simulink model "Basic"  (R2022b)
settings: configuration reference "ERT" (kept outside this file)
PreLoadFcn:
  | %rtwdemo_pmsmfoc_data
StartFcn:
  | %clear executionProfile
StopFcn:
  | %try
  | %  AddExecutionProfileToDataInspector();
  | %end
undefined symbols (not defined in the file or in its folder): bSetOfsAlMdl_C, bSetOfsAlOvrd_C, bUseFrqStrSyntMdl_C, bUseFrqStrSyntOvrd_C, ctrlModeMdl_C, ctrlModeOvrd_C, cTrqSlopeMaxMdl_C, cTrqSlopeMaxOvrd_C, flgInvrCanActvnCmdMdl_C, flgInvrCanActvnCmdOvrd_C, FrqStrSetPMdl_C, FrqStrSetPOvrd_C, IdcMaxMdl_C, IdcMaxOvrd_C, iDCmdMdl_C, iDCmdOvrd_C, IdcMinMdl_C, IdcMinOvrd_C, iQCmdMdl_C, iQCmdOvrd_C, IsSetPMdl_C, IsSetPOvrd_C, kDmpMdl_C, kDmpOvrd_C, KpHighMdl_C, KpHighOvrd_C, KpLowMdl_C, KpLowOvrd_C, NDeltaBoundMdl_C, NDeltaBoundOvrd_C, NSetPMdl_C, NSetPOvrd_C, OfsAlMdl_C, OfsAlOvrd_C, PumpCtlMdl_C, PumpCtlOvrd_C, stDstCReqMdl_C, stDstCReqOvrd_C, stHvbMaiRlyMdl_C, stHvbMaiRlyOvrd_C, stModeReqMdl_C, stModeReqOvrd_C, TrqDmpLimMdl_C, TrqDmpLimOvrd_C, TrqDmpMaxMdl_C, TrqDmpMaxOvrd_C, TrqMaxMdl_C, TrqMaxOvrd_C, TrqMinMdl_C, TrqMinOvrd_C, TrqPAmaxMdl_C, TrqPAmaxOvrd_C, TrqPAminMdl_C, TrqPAminOvrd_C, TrqSetPMdl_C, TrqSetPOvrd_C, Ts_10ms, Ts_1ms, uAlphaCmdMdl_C, uAlphaCmdOvrd_C ... (+12)
settings Model: Creator=The MathWorks, Inc.  LastModifiedBy=M00039784
settings ConfigSetRef: SourceName=ERT  SourceLocation=Base Workspace

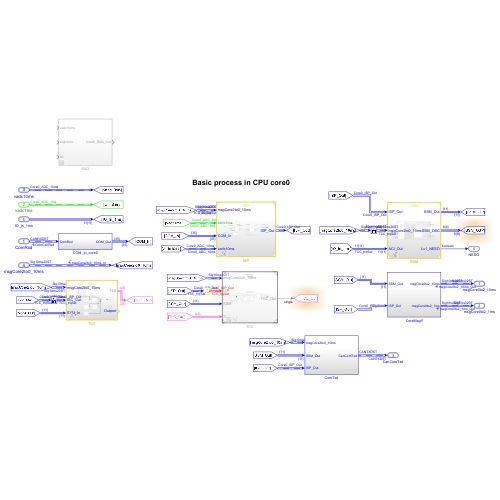
[thumbnail: Simulink's stored preview of the top-level diagram]
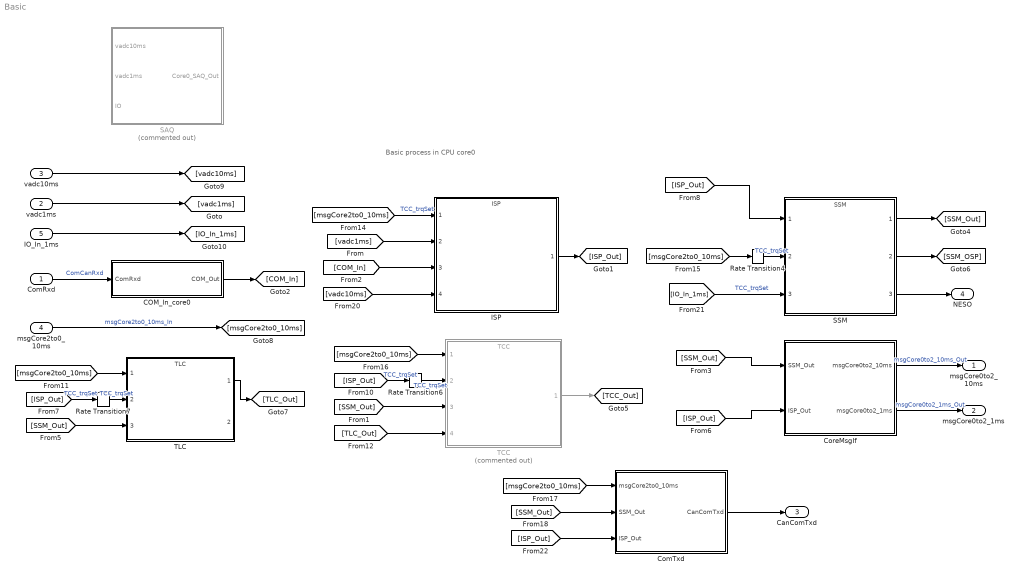
== system Basic ==
  note: Basic process in CPU core0
  ComRxd : Inport  OutDataTypeStr=Bus: CANRXDST  SampleTime=Ts_10ms  BusOutputAsStruct=on
  vadc1ms : Inport  Port=2  OutDataTypeStr=Bus: Core0_ADC_1ms  SampleTime=Ts_1ms  BusOutputAsStruct=on
  vadc10ms : Inport  Port=3  OutDataTypeStr=Bus: Core0_ADC_10ms  SampleTime=Ts_10ms  BusOutputAsStruct=on
  msgCore2to0_10ms : Inport  Port=4  OutDataTypeStr=Bus: Sig10ms20ST  SampleTime=Ts_10ms  BusOutputAsStruct=on
  IO_In_1ms : Inport  Port=5  OutDataTypeStr=Bus: IO_In_1ms
  COM_In_core0 : Subsystem
  ComTxd : Subsystem
  CoreMsgIf : Subsystem
  ISP : ModelReference  ModelNameDialog=ISP.slx  SimulationMode=Normal  ModelReferenceVersion=1.15
  Rate Transition4 : RateTransition  Deterministic=off
  Rate Transition6 : RateTransition  Deterministic=off
  Rate Transition7 : RateTransition  Deterministic=off
  SAQ : Subsystem  Commented=on
  SSM : ModelReference  ModelNameDialog=SSM.slx  SimulationMode=Normal  ModelReferenceVersion=1.14
  TCC : ModelReference  Commented=on  ModelNameDialog=TCC.slx  SimulationMode=Normal  ModelReferenceVersion=1.4
  TLC : ModelReference  ModelNameDialog=TLC.slx  SimulationMode=Normal  ModelReferenceVersion=1.7
  msgCore0to2_10ms : Outport  OutDataTypeStr=Bus: Sig10ms02ST  VectorParamsAs1DForOutWhenUnconnected=off
  msgCore0to2_1ms : Outport  Port=2  OutDataTypeStr=Bus: Sig1ms02ST  VectorParamsAs1DForOutWhenUnconnected=off
  CanComTxd : Outport  Port=3  OutDataTypeStr=Bus: CANTXDST  SampleTime=Ts_10ms  VectorParamsAs1DForOutWhenUnconnected=off
  NESO : Outport  Port=4  SampleTime=Ts_10ms  VectorParamsAs1DForOutWhenUnconnected=off
  wires:
  ComRxd/1 -> COM_In_core0/1(ComRxd)  "ComCanRxd"
  COM_In_core0/1(COM_Out) -> [COM_In]
  SSM/1 -> [SSM_Out]
  [SSM_Out] -> TLC/3
  TLC/1 -> [TLC_Out]
  [TLC_Out] -> TCC/4
  [SSM_Out] -> TCC/3
  TCC/1 -> [TCC_Out]
  [COM_In] -> ISP/3
  [SSM_Out] -> CoreMsgIf/1(SSM_Out)
  [ISP_Out] -> CoreMsgIf/2(ISP_Out)
  CoreMsgIf/1(msgCore0to2_10ms) -> msgCore0to2_10ms/1  "msgCore0to2_10ms_Out"
  CoreMsgIf/2(msgCore0to2_1ms) -> msgCore0to2_1ms/1  "msgCore0to2_1ms_Out"
  SSM/2 -> [SSM_OSP]
  msgCore2to0_10ms/1 -> [msgCore2to0_10ms]  "msgCore2to0_10ms_In"
  [msgCore2to0_10ms] -> TLC/1
  [msgCore2to0_10ms] -> Rate Transition4/1
  [msgCore2to0_10ms] -> TCC/1
  SSM/3 -> NESO/1
  [msgCore2to0_10ms] -> ComTxd/1(msgCore2to0_10ms)
  [SSM_Out] -> ComTxd/2(SSM_Out)
  [ISP_Out] -> ComTxd/3(ISP_Out)
  ComTxd/1(CanComTxd) -> CanComTxd/1
  [msgCore2to0_10ms] -> ISP/1  "TCC_trqSet"
  [ISP_Out] -> Rate Transition7/1  "TCC_trqSet"
  [ISP_Out] -> Rate Transition6/1  "TCC_trqSet"
  ISP/1 -> [ISP_Out]
  Rate Transition4/1 -> SSM/2  "TCC_trqSet"
  Rate Transition6/1 -> TCC/2  "TCC_trqSet"
  Rate Transition7/1 -> TLC/2  "TCC_trqSet"
  vadc10ms/1 -> [vadc10ms]
  IO_In_1ms/1 -> [IO_In_1ms]
  vadc1ms/1 -> [vadc1ms]
  [vadc1ms] -> ISP/2
  [vadc10ms] -> ISP/4
  [ISP_Out] -> SSM/1
  [IO_In_1ms] -> SSM/3  "TCC_trqSet"

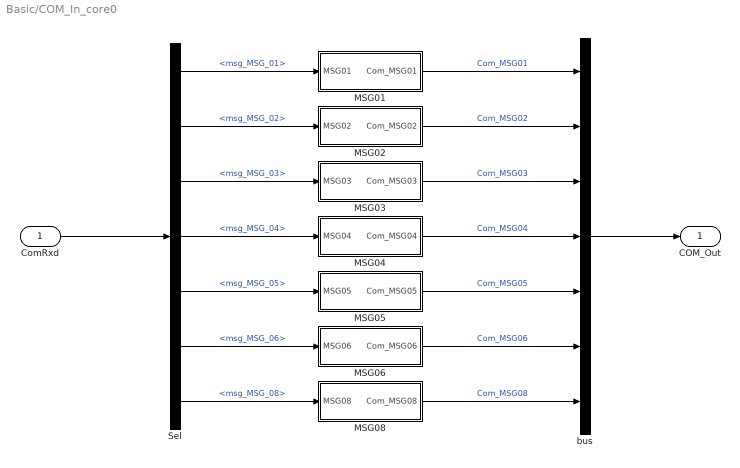
== system Basic/COM_In_core0 ==
  ComRxd : Inport  OutDataTypeStr=Bus: CANRXDST
  MSG01 : Subsystem
  MSG02 : Subsystem
  MSG03 : Subsystem
  MSG04 : Subsystem
  MSG05 : Subsystem
  MSG06 : Subsystem
  MSG08 : Subsystem
  Sel : BusSelector  OutputSignals=msg_MSG_01,msg_MSG_02,msg_MSG_03,msg_MSG_04,msg_MSG_05,msg_MSG_06,msg_MSG_08
  bus : BusCreator  Inputs=7  OutDataTypeStr=Bus: Core0_COM_Out
  COM_Out : Outport  OutDataTypeStr=Bus: Core0_COM_Out  VectorParamsAs1DForOutWhenUnconnected=off
  wires:
  ComRxd/1 -> Sel/1
  bus/1 -> COM_Out/1
  Sel/1 -> MSG01/1(MSG01)  "<msg_MSG_01>"
  MSG01/1(Com_MSG01) -> bus/1  "Com_MSG01"
  Sel/2 -> MSG02/1(MSG02)  "<msg_MSG_02>"
  MSG02/1(Com_MSG02) -> bus/2  "Com_MSG02"
  Sel/3 -> MSG03/1(MSG03)  "<msg_MSG_03>"
  MSG03/1(Com_MSG03) -> bus/3  "Com_MSG03"
  Sel/4 -> MSG04/1(MSG04)  "<msg_MSG_04>"
  MSG04/1(Com_MSG04) -> bus/4  "Com_MSG04"
  Sel/5 -> MSG05/1(MSG05)  "<msg_MSG_05>"
  MSG05/1(Com_MSG05) -> bus/5  "Com_MSG05"
  Sel/6 -> MSG06/1(MSG06)  "<msg_MSG_06>"
  MSG06/1(Com_MSG06) -> bus/6  "Com_MSG06"
  Sel/7 -> MSG08/1(MSG08)  "<msg_MSG_08>"
  MSG08/1(Com_MSG08) -> bus/7  "Com_MSG08"

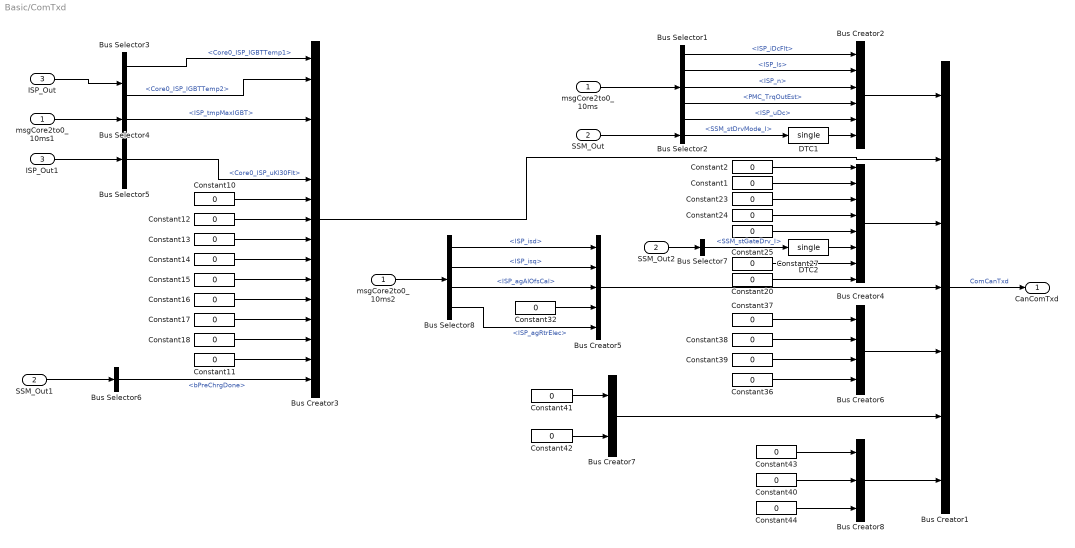
== system Basic/ComTxd ==
  msgCore2to0_10ms : Inport  OutDataTypeStr=Bus: Sig10ms20ST
  SSM_Out : Inport  Port=2  OutDataTypeStr=Bus: Core0_SSM_Out
  ISP_Out : Inport  Port=3  OutDataTypeStr=Bus: Core0_ISP_Out
  Bus Creator1 : BusCreator  Inputs=7  OutDataTypeStr=Bus: CANTXDST  NonVirtualBus=on
  Bus Creator2 : BusCreator  Inputs=6  OutDataTypeStr=Bus: msg_EM_01
  Bus Creator3 : BusCreator  Inputs=17  OutDataTypeStr=Bus: msg_EM_02
  Bus Creator4 : BusCreator  Inputs=8  OutDataTypeStr=Bus: msg_EM_03
  Bus Creator5 : BusCreator  Inputs=5  OutDataTypeStr=Bus: msg_EM_04
  Bus Creator6 : BusCreator  Inputs=4  OutDataTypeStr=Bus: msg_EM_05
  Bus Creator7 : BusCreator  Inputs=2  OutDataTypeStr=Bus: msg_EM_06
  Bus Creator8 : BusCreator  Inputs=3  OutDataTypeStr=Bus: msg_EM_07
  Bus Selector1 : BusSelector  OutputSignals=ISP_iDcFlt,ISP_Is,ISP_n,PMC_TrqOutEst,ISP_uDc
  Bus Selector2 : BusSelector  OutputSignals=SSM_stDrvMode_I
  Bus Selector3 : BusSelector  OutputSignals=Core0_ISP_AnaOut.Core0_ISP_tInvx.Core0_tInv.Core0_ISP_IGBTTemp1,Core0_ISP_AnaOut.Core0_ISP_tInvx.Core0_tInv.Core0_ISP_IGBTTemp2
  Bus Selector4 : BusSelector  OutputSignals=ISP_tmpMaxIGBT
  Bus Selector5 : BusSelector  OutputSignals=Core0_ISP_AnaOut.Core0_ISP_uKl30Flt
  Bus Selector6 : BusSelector  OutputSignals=bPreChrgDone
  Bus Selector7 : BusSelector  OutputSignals=SSM_stGateDrv_I
  Bus Selector8 : BusSelector  OutputSignals=ISP_isd,ISP_isq,ISP_agAlOfsCal,ISP_agRtrElec
  Constant{1..2,20,23..25,27,32,36..44} (17 alike) : Constant  Value=0  OutDataTypeStr=single
  Constant{10..18} (9 alike) : Constant  Value=0  OutDataTypeStr=boolean
  DTC1 : DataTypeConversion  OutDataTypeStr=single  SaturateOnIntegerOverflow=off  RndMeth=Floor
  DTC2 : DataTypeConversion  OutDataTypeStr=single  SaturateOnIntegerOverflow=off  RndMeth=Floor
  ISP_Out1 : InportShadow  Port=3  OutDataTypeStr=Bus: Core0_ISP_Out
  SSM_Out1 : InportShadow  Port=2  OutDataTypeStr=Bus: Core0_SSM_Out
  SSM_Out2 : InportShadow  Port=2  OutDataTypeStr=Bus: Core0_SSM_Out
  msgCore2to0_10ms1 : InportShadow  OutDataTypeStr=Bus: Sig10ms20ST
  msgCore2to0_10ms2 : InportShadow  OutDataTypeStr=Bus: Sig10ms20ST
  CanComTxd : Outport  OutDataTypeStr=Bus: CANTXDST  SampleTime=Ts_10ms  VectorParamsAs1DForOutWhenUnconnected=off
  wires:
  Bus Creator1/1 -> CanComTxd/1  "ComCanTxd"
  msgCore2to0_10ms/1 -> Bus Selector1/1
  Bus Creator2/1 -> Bus Creator1/1
  Bus Selector1/1 -> Bus Creator2/1  "<ISP_iDcFlt>"
  Bus Selector1/2 -> Bus Creator2/2  "<ISP_Is>"
  Bus Selector1/3 -> Bus Creator2/3  "<ISP_n>"
  Bus Creator3/1 -> Bus Creator1/2
  Bus Creator4/1 -> Bus Creator1/3
  Bus Creator5/1 -> Bus Creator1/4
  Bus Creator6/1 -> Bus Creator1/5
  Bus Creator7/1 -> Bus Creator1/6
  Bus Creator8/1 -> Bus Creator1/7
  Bus Selector2/1 -> DTC1/1  "<SSM_stDrvMode_I>"
  Bus Selector3/1 -> Bus Creator3/1  "<Core0_ISP_IGBTTemp1>"
  Bus Selector3/2 -> Bus Creator3/2  "<Core0_ISP_IGBTTemp2>"
  Bus Selector4/1 -> Bus Creator3/4  "<ISP_tmpMaxIGBT>"
  Constant10/1 -> Bus Creator3/8
  Constant18/1 -> Bus Creator3/15
  Constant16/1 -> Bus Creator3/13
  Constant11/1 -> Bus Creator3/16
  Constant12/1 -> Bus Creator3/9
  Constant13/1 -> Bus Creator3/10
  Constant14/1 -> Bus Creator3/11
  Constant15/1 -> Bus Creator3/12
  Constant17/1 -> Bus Creator3/14
  Bus Selector6/1 -> Bus Creator3/17  "<bPreChrgDone>"
  Constant2/1 -> Bus Creator4/1
  Constant1/1 -> Bus Creator4/2
  Constant23/1 -> Bus Creator4/3
  Constant24/1 -> Bus Creator4/4
  Constant25/1 -> Bus Creator4/5
  DTC2/1 -> Bus Creator4/6
  Constant27/1 -> Bus Creator4/7
  Constant20/1 -> Bus Creator4/8
  Bus Selector8/1 -> Bus Creator5/1  "<ISP_isd>"
  Bus Selector8/3 -> Bus Creator5/3  "<ISP_agAlOfsCal>"
  Bus Selector8/2 -> Bus Creator5/2  "<ISP_isq>"
  Bus Selector8/4 -> Bus Creator5/5  "<ISP_agRtrElec>"
  Constant32/1 -> Bus Creator5/4
  Constant37/1 -> Bus Creator6/1
  Constant38/1 -> Bus Creator6/2
  Constant39/1 -> Bus Creator6/3
  Constant36/1 -> Bus Creator6/4
  Constant41/1 -> Bus Creator7/1
  Constant42/1 -> Bus Creator7/2
  Constant44/1 -> Bus Creator8/3
  Constant40/1 -> Bus Creator8/2
  Constant43/1 -> Bus Creator8/1
  Bus Selector1/4 -> Bus Creator2/4  "<PMC_TrqOutEst>"
  Bus Selector1/5 -> Bus Creator2/5  "<ISP_uDc>"
  SSM_Out/1 -> Bus Selector2/1
  DTC1/1 -> Bus Creator2/6
  ISP_Out/1 -> Bus Selector3/1
  msgCore2to0_10ms1/1 -> Bus Selector4/1
  ISP_Out1/1 -> Bus Selector5/1
  SSM_Out1/1 -> Bus Selector6/1
  SSM_Out2/1 -> Bus Selector7/1
  Bus Selector7/1 -> DTC2/1  "<SSM_stGateDrv_I>"
  msgCore2to0_10ms2/1 -> Bus Selector8/1
  Bus Selector5/1 -> Bus Creator3/7  "<Core0_ISP_uKl30Flt>"

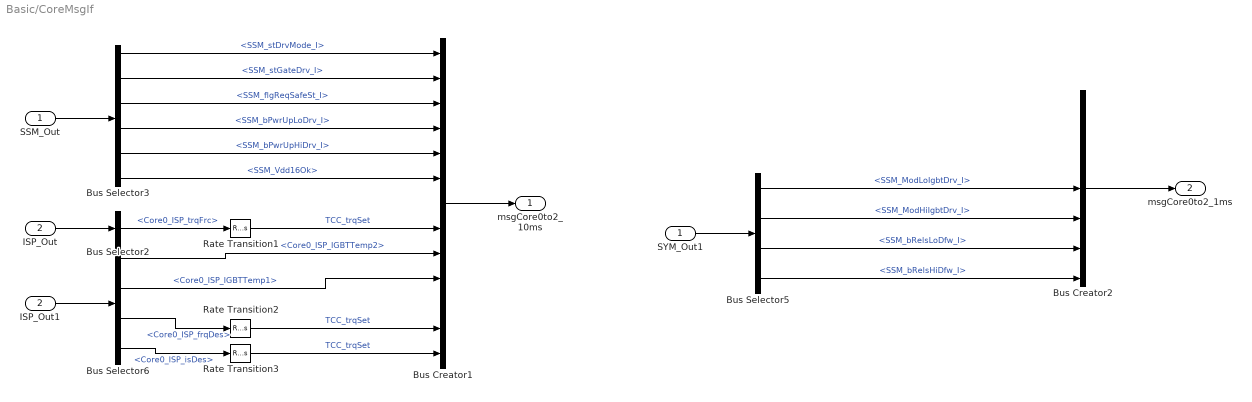
== system Basic/CoreMsgIf ==
  SSM_Out : Inport  OutDataTypeStr=Bus: Core0_SSM_Out
  ISP_Out : Inport  Port=2  OutDataTypeStr=Bus: Core0_ISP_Out
  Bus Creator1 : BusCreator  Inputs=13  OutDataTypeStr=Bus: Sig10ms02ST  NonVirtualBus=on
      settings: InheritFromInputs=off
  Bus Creator2 : BusCreator  Inputs=7  OutDataTypeStr=Bus: Sig1ms02ST  NonVirtualBus=on
      settings: InheritFromInputs=off
  Bus Selector2 : BusSelector  OutputSignals=Core0_ISP_ComCmd.Core0_ISP_trqx.Core0_ISP_trqFrc
  Bus Selector3 : BusSelector  OutputSignals=SSM_stDrvMode_I,SSM_stGateDrv_I,SSM_flgReqSafeSt_I,SSM_bPwrUpLoDrv_I,SSM_bPwrUpHiDrv_I,SSM_Vdd16Ok
  Bus Selector5 : BusSelector  OutputSignals=SSM_ModLoIgbtDrv_I,SSM_ModHiIgbtDrv_I,SSM_bRelsLoDfw_I,SSM_bRelsHiDfw_I
  Bus Selector6 : BusSelector  OutputSignals=Core0_ISP_AnaOut.Core0_ISP_tInvx.Core0_tInv.Core0_ISP_IGBTTemp2,Core0_ISP_AnaOut.Core0_ISP_tInvx.Core0_tInv.Core0_ISP_IGBTTemp1,Core0_ISP_ComCmd.Core0_ISP_cmdx.Core0_ISP_frqDes,Core0_ISP_ComCmd.Core0_ISP_cmdx.Core0_ISP_isDes
  ISP_Out1 : InportShadow  Port=2  OutDataTypeStr=Bus: Core0_ISP_Out
  Rate Transition1 : RateTransition  Deterministic=off  OutPortSampleTime=Ts_10ms
  Rate Transition2 : RateTransition  Deterministic=off  OutPortSampleTime=Ts_10ms
  Rate Transition3 : RateTransition  Deterministic=off  OutPortSampleTime=Ts_10ms
  SYM_Out1 : InportShadow  OutDataTypeStr=Bus: Core0_SSM_Out
  msgCore0to2_10ms : Outport  OutDataTypeStr=Bus: Sig10ms02ST  VectorParamsAs1DForOutWhenUnconnected=off
  msgCore0to2_1ms : Outport  Port=2  OutDataTypeStr=Bus: Sig1ms02ST  VectorParamsAs1DForOutWhenUnconnected=off
  wires:
  Bus Selector3/1 -> Bus Creator1/1  "<SSM_stDrvMode_I>"
  Bus Selector3/2 -> Bus Creator1/2  "<SSM_stGateDrv_I>"
  Bus Creator1/1 -> msgCore0to2_10ms/1
  SSM_Out/1 -> Bus Selector3/1
  Bus Selector2/1 -> Rate Transition1/1  "<Core0_ISP_trqFrc>"
  Bus Selector3/3 -> Bus Creator1/3  "<SSM_flgReqSafeSt_I>"
  ISP_Out/1 -> Bus Selector2/1
  Bus Creator2/1 -> msgCore0to2_1ms/1
  Bus Selector3/4 -> Bus Creator1/4  "<SSM_bPwrUpLoDrv_I>"
  Bus Selector3/5 -> Bus Creator1/5  "<SSM_bPwrUpHiDrv_I>"
  SYM_Out1/1 -> Bus Selector5/1
  Bus Selector5/1 -> Bus Creator2/4  "<SSM_ModLoIgbtDrv_I>"
  Bus Selector5/2 -> Bus Creator2/5  "<SSM_ModHiIgbtDrv_I>"
  Bus Selector5/3 -> Bus Creator2/6  "<SSM_bRelsLoDfw_I>"
  Bus Selector5/4 -> Bus Creator2/7  "<SSM_bRelsHiDfw_I>"
  ISP_Out1/1 -> Bus Selector6/1
  Bus Selector6/1 -> Bus Creator1/9  "<Core0_ISP_IGBTTemp2>"
  Bus Selector6/2 -> Bus Creator1/10  "<Core0_ISP_IGBTTemp1>"
  Bus Selector3/6 -> Bus Creator1/6  "<SSM_Vdd16Ok>"
  Bus Selector6/3 -> Rate Transition2/1  "<Core0_ISP_frqDes>"
  Bus Selector6/4 -> Rate Transition3/1  "<Core0_ISP_isDes>"
  Rate Transition1/1 -> Bus Creator1/8  "TCC_trqSet"
  Rate Transition2/1 -> Bus Creator1/12  "TCC_trqSet"
  Rate Transition3/1 -> Bus Creator1/13  "TCC_trqSet"

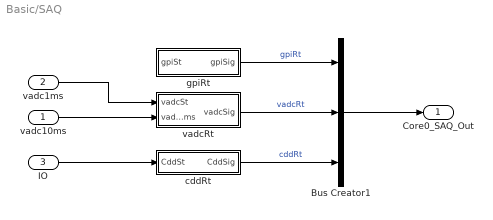
== system Basic/SAQ ==
  vadc10ms : Inport  OutDataTypeStr=Bus: Core0_ADC_10ms
  vadc1ms : Inport  Port=2  OutDataTypeStr=Bus: Core0_ADC_1ms
  IO : Inport  Port=3  OutDataTypeStr=Bus: IO_In_1ms
  Bus Creator1 : BusCreator  Inputs=3  OutDataTypeStr=Bus: Core0_SAQ_Out  NonVirtualBus=on
  cddRt : Subsystem
  gpiRt : Subsystem
  vadcRt : Subsystem
  Core0_SAQ_Out : Outport  OutDataTypeStr=Bus: Core0_SAQ_Out  VectorParamsAs1DForOutWhenUnconnected=off
      settings: AttributesFormatString=Disable Action: %<OutputWhenDisabled>
  wires:
  Bus Creator1/1 -> Core0_SAQ_Out/1
  gpiRt/1(gpiSig) -> Bus Creator1/1  "gpiRt"
  vadc10ms/1 -> vadcRt/2(vadc10ms)
  vadc1ms/1 -> vadcRt/1(vadcSt)
  vadcRt/1(vadcSig) -> Bus Creator1/2  "vadcRt"
  IO/1 -> cddRt/1(CddSt)
  cddRt/1(CddSig) -> Bus Creator1/3  "cddRt"

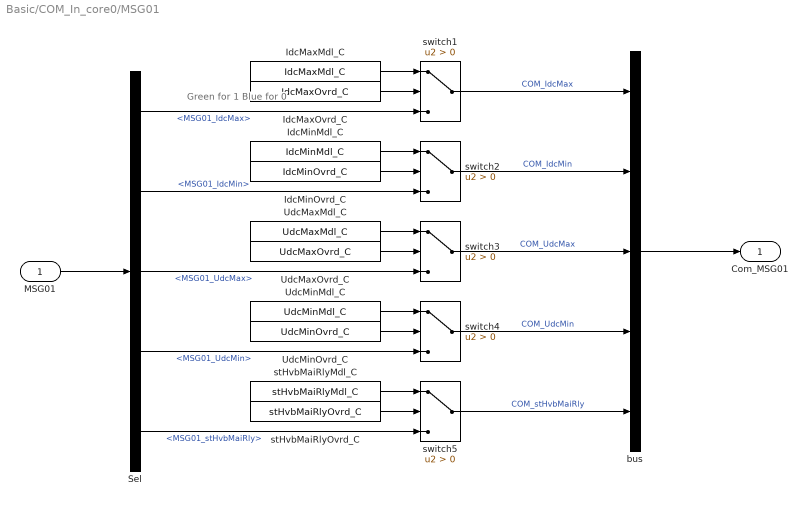
== system Basic/COM_In_core0/MSG01 ==
  note: Green  for 1
      | Blue  for 0
  MSG01 : Inport
  IdcMaxMdl_C : Constant  Value=IdcMaxMdl_C
      mask Display:
      | tmpx = get_param(gcbh,'Value');
      | a= evalin('base',[tmpx,'.Value;']);
      | disp([tmpx,': ',num2str(a)]);
  IdcMaxOvrd_C : Constant  Value=IdcMaxOvrd_C
      mask Display:
      | tmpx = get_param(gcbh,'Value');
      | a= evalin('base',[tmpx,'.Value;']);
      | if a==0
      |     color('blue');
      | else
      |     color('green');
      | end
      | disp([tmpx,': ',num2str(a)]);
  IdcMinMdl_C : Constant  Value=IdcMinMdl_C
      mask Display:
      | tmpx = get_param(gcbh,'Value');
      | a= evalin('base',[tmpx,'.Value;']);
      | disp([tmpx,': ',num2str(a)]);
  IdcMinOvrd_C : Constant  Value=IdcMinOvrd_C
      mask Display:
      | tmpx = get_param(gcbh,'Value');
      | a= evalin('base',[tmpx,'.Value;']);
      | if a==0
      |     color('red');
      | else
      |     color('green');
      | end
      | disp([tmpx,': ',num2str(a)]);
  Sel : BusSelector  OutputSignals=MSG01_IdcMax,MSG01_IdcMin,MSG01_UdcMax,MSG01_UdcMin,MSG01_stHvbMaiRly
  UdcMaxMdl_C : Constant  Value=UdcMaxMdl_C
      mask Display:
      | tmpx = get_param(gcbh,'Value');
      | a= evalin('base',[tmpx,'.Value;']);
      | disp([tmpx,': ',num2str(a)]);
  UdcMaxOvrd_C : Constant  Value=UdcMaxOvrd_C
      mask Display:
      | tmpx = get_param(gcbh,'Value');
      | a= evalin('base',[tmpx,'.Value;']);
      | if a==0
      |     color('blue');
      | else
      |     color('green');
      | end
      | disp([tmpx,': ',num2str(a)]);
  UdcMinMdl_C : Constant  Value=UdcMinMdl_C
      mask Display:
      | tmpx = get_param(gcbh,'Value');
      | a= evalin('base',[tmpx,'.Value;']);
      | disp([tmpx,': ',num2str(a)]);
  UdcMinOvrd_C : Constant  Value=UdcMinOvrd_C
      mask Display:
      | tmpx = get_param(gcbh,'Value');
      | a= evalin('base',[tmpx,'.Value;']);
      | if a==0
      |     color('blue');
      | else
      |     color('green');
      | end
      | disp([tmpx,': ',num2str(a)]);
  bus : BusCreator  Inputs=5
  stHvbMaiRlyMdl_C : Constant  Value=stHvbMaiRlyMdl_C
      mask Display:
      | tmpx = get_param(gcbh,'Value');
      | a= evalin('base',[tmpx,'.Value;']);
      | disp([tmpx,': ',num2str(a)]);
  stHvbMaiRlyOvrd_C : Constant  Value=stHvbMaiRlyOvrd_C
      mask Display:
      | tmpx = get_param(gcbh,'Value');
      | a= evalin('base',[tmpx,'.Value;']);
      | if a==0
      |     color('blue');
      | else
      |     color('green');
      | end
      | disp([tmpx,': ',num2str(a)]);
  switch{1..5} (5 alike) : Switch  Criteria=u2 > Threshold  SaturateOnIntegerOverflow=off  InputSameDT=off
  Com_MSG01 : Outport  VectorParamsAs1DForOutWhenUnconnected=off
  wires:
  MSG01/1 -> Sel/1
  bus/1 -> Com_MSG01/1
  IdcMaxOvrd_C/1 -> switch1/2
  IdcMaxMdl_C/1 -> switch1/1
  switch1/1 -> bus/1  "COM_IdcMax"
  Sel/1 -> switch1/3  "<MSG01_IdcMax>"
  IdcMinOvrd_C/1 -> switch2/2
  IdcMinMdl_C/1 -> switch2/1
  switch2/1 -> bus/2  "COM_IdcMin"
  Sel/2 -> switch2/3  "<MSG01_IdcMin>"
  UdcMaxOvrd_C/1 -> switch3/2
  UdcMaxMdl_C/1 -> switch3/1
  switch3/1 -> bus/3  "COM_UdcMax"
  Sel/3 -> switch3/3  "<MSG01_UdcMax>"
  UdcMinOvrd_C/1 -> switch4/2
  UdcMinMdl_C/1 -> switch4/1
  switch4/1 -> bus/4  "COM_UdcMin"
  Sel/4 -> switch4/3  "<MSG01_UdcMin>"
  stHvbMaiRlyOvrd_C/1 -> switch5/2
  stHvbMaiRlyMdl_C/1 -> switch5/1
  switch5/1 -> bus/5  "COM_stHvbMaiRly"
  Sel/5 -> switch5/3  "<MSG01_stHvbMaiRly>"

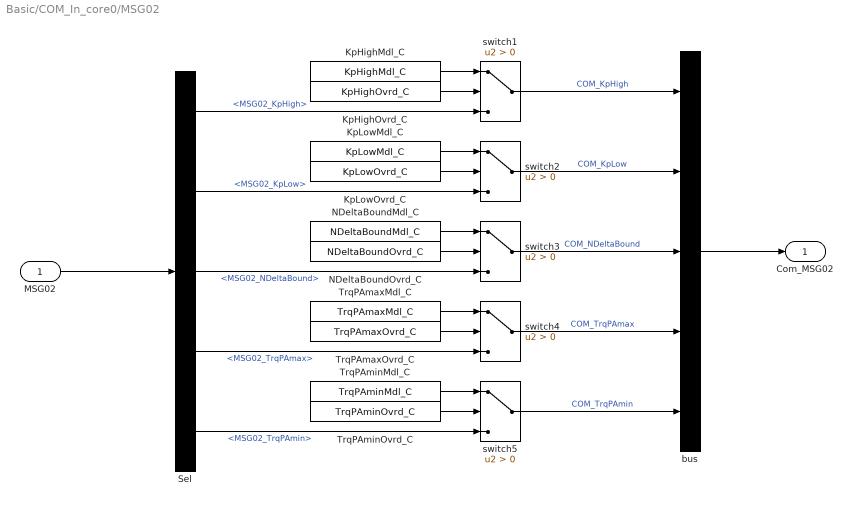
== system Basic/COM_In_core0/MSG02 ==
  MSG02 : Inport
  KpHighMdl_C : Constant  Value=KpHighMdl_C
      mask Display:
      | tmpx = get_param(gcbh,'Value');
      | a= evalin('base',[tmpx,'.Value;']);
      | disp([tmpx,': ',num2str(a)]);
  KpHighOvrd_C : Constant  Value=KpHighOvrd_C
      mask Display:
      | tmpx = get_param(gcbh,'Value');
      | a= evalin('base',[tmpx,'.Value;']);
      | if a==0
      |     color('blue');
      | else
      |     color('green');
      | end
      | disp([tmpx,': ',num2str(a)]);
  KpLowMdl_C : Constant  Value=KpLowMdl_C
      mask Display:
      | tmpx = get_param(gcbh,'Value');
      | a= evalin('base',[tmpx,'.Value;']);
      | disp([tmpx,': ',num2str(a)]);
  KpLowOvrd_C : Constant  Value=KpLowOvrd_C
      mask Display:
      | tmpx = get_param(gcbh,'Value');
      | a= evalin('base',[tmpx,'.Value;']);
      | if a==0
      |     color('blue');
      | else
      |     color('green');
      | end
      | disp([tmpx,': ',num2str(a)]);
  NDeltaBoundMdl_C : Constant  Value=NDeltaBoundMdl_C
      mask Display:
      | tmpx = get_param(gcbh,'Value');
      | a= evalin('base',[tmpx,'.Value;']);
      | disp([tmpx,': ',num2str(a)]);
  NDeltaBoundOvrd_C : Constant  Value=NDeltaBoundOvrd_C
      mask Display:
      | tmpx = get_param(gcbh,'Value');
      | a= evalin('base',[tmpx,'.Value;']);
      | if a==0
      |     color('blue');
      | else
      |     color('green');
      | end
      | disp([tmpx,': ',num2str(a)]);
  Sel : BusSelector  OutputSignals=MSG02_KpHigh,MSG02_KpLow,MSG02_NDeltaBound,MSG02_TrqPAmax,MSG02_TrqPAmin
  TrqPAmaxMdl_C : Constant  Value=TrqPAmaxMdl_C
      mask Display:
      | tmpx = get_param(gcbh,'Value');
      | a= evalin('base',[tmpx,'.Value;']);
      | disp([tmpx,': ',num2str(a)]);
  TrqPAmaxOvrd_C : Constant  Value=TrqPAmaxOvrd_C
      mask Display:
      | tmpx = get_param(gcbh,'Value');
      | a= evalin('base',[tmpx,'.Value;']);
      | if a==0
      |     color('blue');
      | else
      |     color('green');
      | end
      | disp([tmpx,': ',num2str(a)]);
  TrqPAminMdl_C : Constant  Value=TrqPAminMdl_C
      mask Display:
      | tmpx = get_param(gcbh,'Value');
      | a= evalin('base',[tmpx,'.Value;']);
      | disp([tmpx,': ',num2str(a)]);
  TrqPAminOvrd_C : Constant  Value=TrqPAminOvrd_C
      mask Display:
      | tmpx = get_param(gcbh,'Value');
      | a= evalin('base',[tmpx,'.Value;']);
      | if a==0
      |     color('blue');
      | else
      |     color('green');
      | end
      | disp([tmpx,': ',num2str(a)]);
  bus : BusCreator  Inputs=5  OutDataTypeStr=Bus: Com_MSG02
  switch{1..5} (5 alike) : Switch  Criteria=u2 > Threshold  SaturateOnIntegerOverflow=off  InputSameDT=off
  Com_MSG02 : Outport  VectorParamsAs1DForOutWhenUnconnected=off
  wires:
  MSG02/1 -> Sel/1
  bus/1 -> Com_MSG02/1
  KpHighOvrd_C/1 -> switch1/2
  KpHighMdl_C/1 -> switch1/1
  switch1/1 -> bus/1  "COM_KpHigh"
  Sel/1 -> switch1/3  "<MSG02_KpHigh>"
  KpLowOvrd_C/1 -> switch2/2
  KpLowMdl_C/1 -> switch2/1
  switch2/1 -> bus/2  "COM_KpLow"
  Sel/2 -> switch2/3  "<MSG02_KpLow>"
  NDeltaBoundOvrd_C/1 -> switch3/2
  NDeltaBoundMdl_C/1 -> switch3/1
  switch3/1 -> bus/3  "COM_NDeltaBound"
  Sel/3 -> switch3/3  "<MSG02_NDeltaBound>"
  TrqPAmaxOvrd_C/1 -> switch4/2
  TrqPAmaxMdl_C/1 -> switch4/1
  switch4/1 -> bus/4  "COM_TrqPAmax"
  Sel/4 -> switch4/3  "<MSG02_TrqPAmax>"
  TrqPAminOvrd_C/1 -> switch5/2
  TrqPAminMdl_C/1 -> switch5/1
  switch5/1 -> bus/5  "COM_TrqPAmin"
  Sel/5 -> switch5/3  "<MSG02_TrqPAmin>"

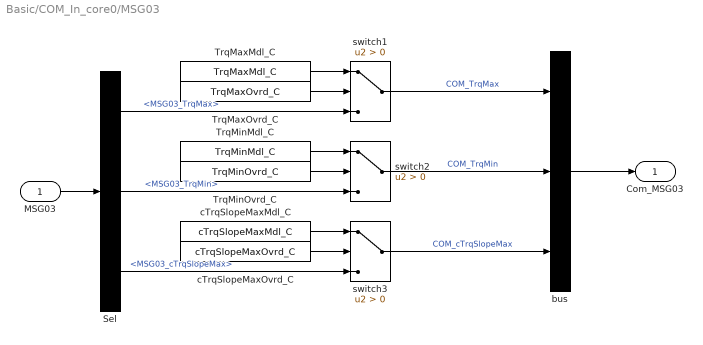
== system Basic/COM_In_core0/MSG03 ==
  MSG03 : Inport
  Sel : BusSelector  OutputSignals=MSG03_TrqMax,MSG03_TrqMin,MSG03_cTrqSlopeMax
  TrqMaxMdl_C : Constant  Value=TrqMaxMdl_C
      mask Display:
      | tmpx = get_param(gcbh,'Value');
      | a= evalin('base',[tmpx,'.Value;']);
      | disp([tmpx,': ',num2str(a)]);
  TrqMaxOvrd_C : Constant  Value=TrqMaxOvrd_C
      mask Display:
      | tmpx = get_param(gcbh,'Value');
      | a= evalin('base',[tmpx,'.Value;']);
      | if a==0
      |     color('blue');
      | else
      |     color('green');
      | end
      | disp([tmpx,': ',num2str(a)]);
  TrqMinMdl_C : Constant  Value=TrqMinMdl_C
      mask Display:
      | tmpx = get_param(gcbh,'Value');
      | a= evalin('base',[tmpx,'.Value;']);
      | disp([tmpx,': ',num2str(a)]);
  TrqMinOvrd_C : Constant  Value=TrqMinOvrd_C
      mask Display:
      | tmpx = get_param(gcbh,'Value');
      | a= evalin('base',[tmpx,'.Value;']);
      | if a==0
      |     color('blue');
      | else
      |     color('green');
      | end
      | disp([tmpx,': ',num2str(a)]);
  bus : BusCreator  Inputs=3  OutDataTypeStr=Bus: Com_MSG03
  cTrqSlopeMaxMdl_C : Constant  Value=cTrqSlopeMaxMdl_C
      mask Display:
      | tmpx = get_param(gcbh,'Value');
      | a= evalin('base',[tmpx,'.Value;']);
      | disp([tmpx,': ',num2str(a)]);
  cTrqSlopeMaxOvrd_C : Constant  Value=cTrqSlopeMaxOvrd_C
      mask Display:
      | tmpx = get_param(gcbh,'Value');
      | a= evalin('base',[tmpx,'.Value;']);
      | if a==0
      |     color('blue');
      | else
      |     color('green');
      | end
      | disp([tmpx,': ',num2str(a)]);
  switch1 : Switch  Criteria=u2 > Threshold  SaturateOnIntegerOverflow=off  InputSameDT=off
  switch2 : Switch  Criteria=u2 > Threshold  SaturateOnIntegerOverflow=off  InputSameDT=off
  switch3 : Switch  Criteria=u2 > Threshold  SaturateOnIntegerOverflow=off  InputSameDT=off
  Com_MSG03 : Outport  VectorParamsAs1DForOutWhenUnconnected=off
  wires:
  MSG03/1 -> Sel/1
  bus/1 -> Com_MSG03/1
  TrqMaxOvrd_C/1 -> switch1/2
  TrqMaxMdl_C/1 -> switch1/1
  switch1/1 -> bus/1  "COM_TrqMax"
  Sel/1 -> switch1/3  "<MSG03_TrqMax>"
  TrqMinOvrd_C/1 -> switch2/2
  TrqMinMdl_C/1 -> switch2/1
  switch2/1 -> bus/2  "COM_TrqMin"
  Sel/2 -> switch2/3  "<MSG03_TrqMin>"
  cTrqSlopeMaxOvrd_C/1 -> switch3/2
  cTrqSlopeMaxMdl_C/1 -> switch3/1
  switch3/1 -> bus/3  "COM_cTrqSlopeMax"
  Sel/3 -> switch3/3  "<MSG03_cTrqSlopeMax>"

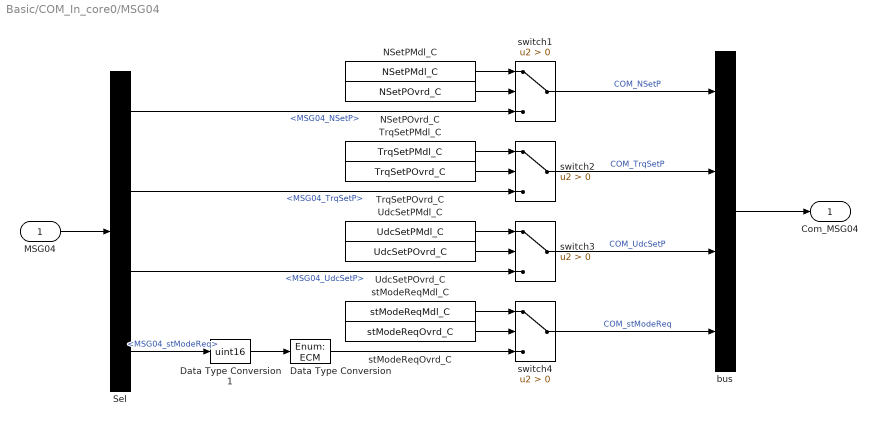
== system Basic/COM_In_core0/MSG04 ==
  MSG04 : Inport
  Data Type Conversion : DataTypeConversion  OutDataTypeStr=Enum: ECM  SaturateOnIntegerOverflow=off  RndMeth=Floor
  Data Type Conversion1 : DataTypeConversion  OutDataTypeStr=uint16  SaturateOnIntegerOverflow=off  RndMeth=Floor
  NSetPMdl_C : Constant  Value=NSetPMdl_C
      mask Display:
      | tmpx = get_param(gcbh,'Value');
      | a= evalin('base',[tmpx,'.Value;']);
      | disp([tmpx,': ',num2str(a)]);
  NSetPOvrd_C : Constant  Value=NSetPOvrd_C
      mask Display:
      | tmpx = get_param(gcbh,'Value');
      | a= evalin('base',[tmpx,'.Value;']);
      | if a==0
      |     color('blue');
      | else
      |     color('green');
      | end
      | disp([tmpx,': ',num2str(a)]);
  Sel : BusSelector  OutputSignals=MSG04_NSetP,MSG04_TrqSetP,MSG04_UdcSetP,MSG04_stModeReq
  TrqSetPMdl_C : Constant  Value=TrqSetPMdl_C
      mask Display:
      | tmpx = get_param(gcbh,'Value');
      | a= evalin('base',[tmpx,'.Value;']);
      | disp([tmpx,': ',num2str(a)]);
  TrqSetPOvrd_C : Constant  Value=TrqSetPOvrd_C
      mask Display:
      | tmpx = get_param(gcbh,'Value');
      | a= evalin('base',[tmpx,'.Value;']);
      | if a==0
      |     color('blue');
      | else
      |     color('green');
      | end
      | disp([tmpx,': ',num2str(a)]);
  UdcSetPMdl_C : Constant  Value=UdcSetPMdl_C
      mask Display:
      | tmpx = get_param(gcbh,'Value');
      | a= evalin('base',[tmpx,'.Value;']);
      | disp([tmpx,': ',num2str(a)]);
  UdcSetPOvrd_C : Constant  Value=UdcSetPOvrd_C
      mask Display:
      | tmpx = get_param(gcbh,'Value');
      | a= evalin('base',[tmpx,'.Value;']);
      | if a==0
      |     color('blue');
      | else
      |     color('green');
      | end
      | disp([tmpx,': ',num2str(a)]);
  bus : BusCreator  Inputs=4  OutDataTypeStr=Bus: Com_MSG04
  stModeReqMdl_C : Constant  Value=stModeReqMdl_C
      mask Display:
      | tmpx = get_param(gcbh,'Value');
      | a= evalin('base',[tmpx,'.Value;']);
      | disp([tmpx,': ',num2str(a)]);
  stModeReqOvrd_C : Constant  Value=stModeReqOvrd_C
      mask Display:
      | tmpx = get_param(gcbh,'Value');
      | a= evalin('base',[tmpx,'.Value;']);
      | if a==0
      |     color('blue');
      | else
      |     color('green');
      | end
      | disp([tmpx,': ',num2str(a)]);
  switch{1..4} (4 alike) : Switch  Criteria=u2 > Threshold  SaturateOnIntegerOverflow=off  InputSameDT=off
  Com_MSG04 : Outport  VectorParamsAs1DForOutWhenUnconnected=off
  wires:
  MSG04/1 -> Sel/1
  bus/1 -> Com_MSG04/1
  NSetPOvrd_C/1 -> switch1/2
  NSetPMdl_C/1 -> switch1/1
  switch1/1 -> bus/1  "COM_NSetP"
  Sel/1 -> switch1/3  "<MSG04_NSetP>"
  TrqSetPOvrd_C/1 -> switch2/2
  TrqSetPMdl_C/1 -> switch2/1
  switch2/1 -> bus/2  "COM_TrqSetP"
  Sel/2 -> switch2/3  "<MSG04_TrqSetP>"
  UdcSetPOvrd_C/1 -> switch3/2
  UdcSetPMdl_C/1 -> switch3/1
  switch3/1 -> bus/3  "COM_UdcSetP"
  Sel/3 -> switch3/3  "<MSG04_UdcSetP>"
  stModeReqOvrd_C/1 -> switch4/2
  stModeReqMdl_C/1 -> switch4/1
  switch4/1 -> bus/4  "COM_stModeReq"
  Sel/4 -> Data Type Conversion1/1  "<MSG04_stModeReq>"
  Data Type Conversion/1 -> switch4/3
  Data Type Conversion1/1 -> Data Type Conversion/1

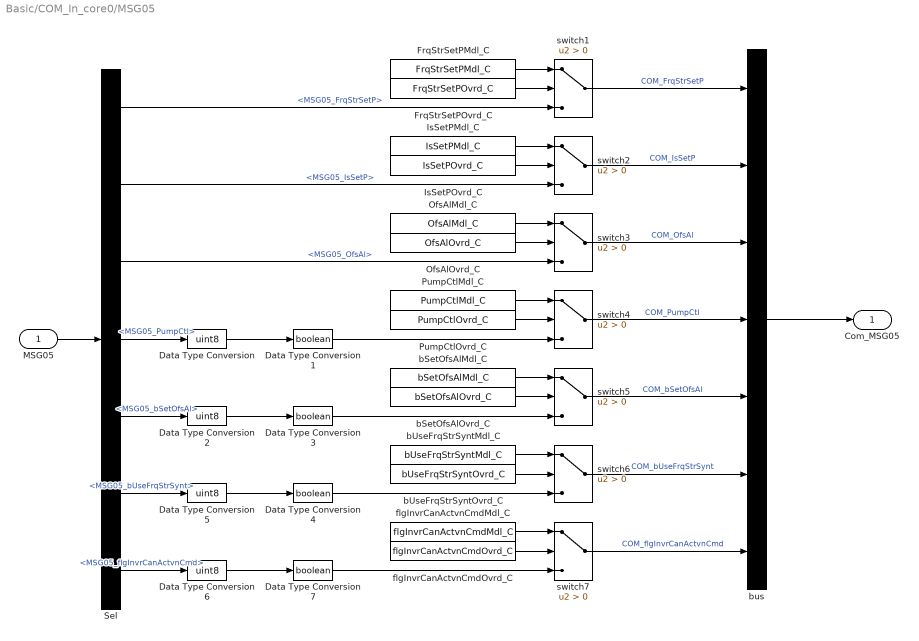
== system Basic/COM_In_core0/MSG05 ==
  MSG05 : Inport
  Data Type Conversion{,2,5..6} (4 alike) : DataTypeConversion  OutDataTypeStr=uint8  SaturateOnIntegerOverflow=off  RndMeth=Floor
  Data Type Conversion{1,3..4,7} (4 alike) : DataTypeConversion  OutDataTypeStr=boolean  SaturateOnIntegerOverflow=off  RndMeth=Floor
  FrqStrSetPMdl_C : Constant  Value=FrqStrSetPMdl_C
      mask Display:
      | tmpx = get_param(gcbh,'Value');
      | a= evalin('base',[tmpx,'.Value;']);
      | disp([tmpx,': ',num2str(a)]);
  FrqStrSetPOvrd_C : Constant  Value=FrqStrSetPOvrd_C
      mask Display:
      | tmpx = get_param(gcbh,'Value');
      | a= evalin('base',[tmpx,'.Value;']);
      | if a==0
      |     color('blue');
      | else
      |     color('green');
      | end
      | disp([tmpx,': ',num2str(a)]);
  IsSetPMdl_C : Constant  Value=IsSetPMdl_C
      mask Display:
      | tmpx = get_param(gcbh,'Value');
      | a= evalin('base',[tmpx,'.Value;']);
      | disp([tmpx,': ',num2str(a)]);
  IsSetPOvrd_C : Constant  Value=IsSetPOvrd_C
      mask Display:
      | tmpx = get_param(gcbh,'Value');
      | a= evalin('base',[tmpx,'.Value;']);
      | if a==0
      |     color('blue');
      | else
      |     color('green');
      | end
      | disp([tmpx,': ',num2str(a)]);
  OfsAlMdl_C : Constant  Value=OfsAlMdl_C
      mask Display:
      | tmpx = get_param(gcbh,'Value');
      | a= evalin('base',[tmpx,'.Value;']);
      | disp([tmpx,': ',num2str(a)]);
  OfsAlOvrd_C : Constant  Value=OfsAlOvrd_C
      mask Display:
      | tmpx = get_param(gcbh,'Value');
      | a= evalin('base',[tmpx,'.Value;']);
      | if a==0
      |     color('blue');
      | else
      |     color('green');
      | end
      | disp([tmpx,': ',num2str(a)]);
  PumpCtlMdl_C : Constant  Value=PumpCtlMdl_C
      mask Display:
      | tmpx = get_param(gcbh,'Value');
      | a= evalin('base',[tmpx,'.Value;']);
      | disp([tmpx,': ',num2str(a)]);
  PumpCtlOvrd_C : Constant  Value=PumpCtlOvrd_C
      mask Display:
      | tmpx = get_param(gcbh,'Value');
      | a= evalin('base',[tmpx,'.Value;']);
      | if a==0
      |     color('blue');
      | else
      |     color('green');
      | end
      | disp([tmpx,': ',num2str(a)]);
  Sel : BusSelector  OutputSignals=MSG05_FrqStrSetP,MSG05_IsSetP,MSG05_OfsAl,MSG05_PumpCtl,MSG05_bSetOfsAl,MSG05_bUseFrqStrSynt,MSG05_flgInvrCanActvnCmd
  bSetOfsAlMdl_C : Constant  Value=bSetOfsAlMdl_C
      mask Display:
      | tmpx = get_param(gcbh,'Value');
      | a= evalin('base',[tmpx,'.Value;']);
      | disp([tmpx,': ',num2str(a)]);
  bSetOfsAlOvrd_C : Constant  Value=bSetOfsAlOvrd_C
      mask Display:
      | tmpx = get_param(gcbh,'Value');
      | a= evalin('base',[tmpx,'.Value;']);
      | if a==0
      |     color('blue');
      | else
      |     color('green');
      | end
      | disp([tmpx,': ',num2str(a)]);
  bUseFrqStrSyntMdl_C : Constant  Value=bUseFrqStrSyntMdl_C
      mask Display:
      | tmpx = get_param(gcbh,'Value');
      | a= evalin('base',[tmpx,'.Value;']);
      | disp([tmpx,': ',num2str(a)]);
  bUseFrqStrSyntOvrd_C : Constant  Value=bUseFrqStrSyntOvrd_C
      mask Display:
      | tmpx = get_param(gcbh,'Value');
      | a= evalin('base',[tmpx,'.Value;']);
      | if a==0
      |     color('blue');
      | else
      |     color('green');
      | end
      | disp([tmpx,': ',num2str(a)]);
  bus : BusCreator  Inputs=7  OutDataTypeStr=Bus: Com_MSG05
  flgInvrCanActvnCmdMdl_C : Constant  Value=flgInvrCanActvnCmdMdl_C
      mask Display:
      | tmpx = get_param(gcbh,'Value');
      | a= evalin('base',[tmpx,'.Value;']);
      | disp([tmpx,': ',num2str(a)]);
  flgInvrCanActvnCmdOvrd_C : Constant  Value=flgInvrCanActvnCmdOvrd_C
      mask Display:
      | tmpx = get_param(gcbh,'Value');
      | a= evalin('base',[tmpx,'.Value;']);
      | if a==0
      |     color('blue');
      | else
      |     color('green');
      | end
      | disp([tmpx,': ',num2str(a)]);
  switch{1..7} (7 alike) : Switch  Criteria=u2 > Threshold  SaturateOnIntegerOverflow=off  InputSameDT=off
  Com_MSG05 : Outport  VectorParamsAs1DForOutWhenUnconnected=off
  wires:
  MSG05/1 -> Sel/1
  bus/1 -> Com_MSG05/1
  FrqStrSetPOvrd_C/1 -> switch1/2
  FrqStrSetPMdl_C/1 -> switch1/1
  switch1/1 -> bus/1  "COM_FrqStrSetP"
  Sel/1 -> switch1/3  "<MSG05_FrqStrSetP>"
  IsSetPOvrd_C/1 -> switch2/2
  IsSetPMdl_C/1 -> switch2/1
  switch2/1 -> bus/2  "COM_IsSetP"
  Sel/2 -> switch2/3  "<MSG05_IsSetP>"
  OfsAlOvrd_C/1 -> switch3/2
  OfsAlMdl_C/1 -> switch3/1
  switch3/1 -> bus/3  "COM_OfsAl"
  Sel/3 -> switch3/3  "<MSG05_OfsAl>"
  PumpCtlOvrd_C/1 -> switch4/2
  PumpCtlMdl_C/1 -> switch4/1
  switch4/1 -> bus/4  "COM_PumpCtl"
  Sel/4 -> Data Type Conversion/1  "<MSG05_PumpCtl>"
  bSetOfsAlOvrd_C/1 -> switch5/2
  bSetOfsAlMdl_C/1 -> switch5/1
  switch5/1 -> bus/5  "COM_bSetOfsAl"
  Sel/5 -> Data Type Conversion2/1  "<MSG05_bSetOfsAl>"
  bUseFrqStrSyntOvrd_C/1 -> switch6/2
  bUseFrqStrSyntMdl_C/1 -> switch6/1
  switch6/1 -> bus/6  "COM_bUseFrqStrSynt"
  Sel/6 -> Data Type Conversion5/1  "<MSG05_bUseFrqStrSynt>"
  flgInvrCanActvnCmdOvrd_C/1 -> switch7/2
  flgInvrCanActvnCmdMdl_C/1 -> switch7/1
  switch7/1 -> bus/7  "COM_flgInvrCanActvnCmd"
  Sel/7 -> Data Type Conversion6/1  "<MSG05_flgInvrCanActvnCmd>"
  Data Type Conversion/1 -> Data Type Conversion1/1
  Data Type Conversion1/1 -> switch4/3
  Data Type Conversion3/1 -> switch5/3
  Data Type Conversion2/1 -> Data Type Conversion3/1
  Data Type Conversion4/1 -> switch6/3
  Data Type Conversion5/1 -> Data Type Conversion4/1
  Data Type Conversion6/1 -> Data Type Conversion7/1
  Data Type Conversion7/1 -> switch7/3

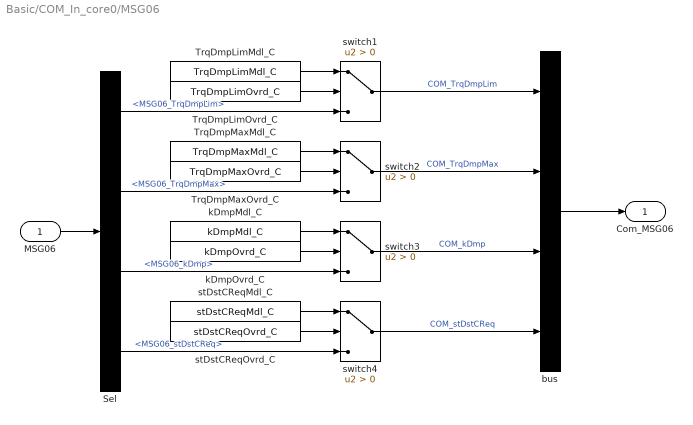
== system Basic/COM_In_core0/MSG06 ==
  MSG06 : Inport
  Sel : BusSelector  OutputSignals=MSG06_TrqDmpLim,MSG06_TrqDmpMax,MSG06_kDmp,MSG06_stDstCReq
  TrqDmpLimMdl_C : Constant  Value=TrqDmpLimMdl_C
      mask Display:
      | tmpx = get_param(gcbh,'Value');
      | a= evalin('base',[tmpx,'.Value;']);
      | disp([tmpx,': ',num2str(a)]);
  TrqDmpLimOvrd_C : Constant  Value=TrqDmpLimOvrd_C
      mask Display:
      | tmpx = get_param(gcbh,'Value');
      | a= evalin('base',[tmpx,'.Value;']);
      | if a==0
      |     color('blue');
      | else
      |     color('green');
      | end
      | disp([tmpx,': ',num2str(a)]);
  TrqDmpMaxMdl_C : Constant  Value=TrqDmpMaxMdl_C
      mask Display:
      | tmpx = get_param(gcbh,'Value');
      | a= evalin('base',[tmpx,'.Value;']);
      | disp([tmpx,': ',num2str(a)]);
  TrqDmpMaxOvrd_C : Constant  Value=TrqDmpMaxOvrd_C
      mask Display:
      | tmpx = get_param(gcbh,'Value');
      | a= evalin('base',[tmpx,'.Value;']);
      | if a==0
      |     color('blue');
      | else
      |     color('green');
      | end
      | disp([tmpx,': ',num2str(a)]);
  bus : BusCreator  Inputs=4  OutDataTypeStr=Bus: Com_MSG06
  kDmpMdl_C : Constant  Value=kDmpMdl_C
      mask Display:
      | tmpx = get_param(gcbh,'Value');
      | a= evalin('base',[tmpx,'.Value;']);
      | disp([tmpx,': ',num2str(a)]);
  kDmpOvrd_C : Constant  Value=kDmpOvrd_C
      mask Display:
      | tmpx = get_param(gcbh,'Value');
      | a= evalin('base',[tmpx,'.Value;']);
      | if a==0
      |     color('blue');
      | else
      |     color('green');
      | end
      | disp([tmpx,': ',num2str(a)]);
  stDstCReqMdl_C : Constant  Value=stDstCReqMdl_C
      mask Display:
      | tmpx = get_param(gcbh,'Value');
      | a= evalin('base',[tmpx,'.Value;']);
      | disp([tmpx,': ',num2str(a)]);
  stDstCReqOvrd_C : Constant  Value=stDstCReqOvrd_C
      mask Display:
      | tmpx = get_param(gcbh,'Value');
      | a= evalin('base',[tmpx,'.Value;']);
      | if a==0
      |     color('blue');
      | else
      |     color('green');
      | end
      | disp([tmpx,': ',num2str(a)]);
  switch{1..4} (4 alike) : Switch  Criteria=u2 > Threshold  SaturateOnIntegerOverflow=off  InputSameDT=off
  Com_MSG06 : Outport  VectorParamsAs1DForOutWhenUnconnected=off
  wires:
  MSG06/1 -> Sel/1
  bus/1 -> Com_MSG06/1
  TrqDmpLimOvrd_C/1 -> switch1/2
  TrqDmpLimMdl_C/1 -> switch1/1
  switch1/1 -> bus/1  "COM_TrqDmpLim"
  Sel/1 -> switch1/3  "<MSG06_TrqDmpLim>"
  TrqDmpMaxOvrd_C/1 -> switch2/2
  TrqDmpMaxMdl_C/1 -> switch2/1
  switch2/1 -> bus/2  "COM_TrqDmpMax"
  Sel/2 -> switch2/3  "<MSG06_TrqDmpMax>"
  kDmpOvrd_C/1 -> switch3/2
  kDmpMdl_C/1 -> switch3/1
  switch3/1 -> bus/3  "COM_kDmp"
  Sel/3 -> switch3/3  "<MSG06_kDmp>"
  stDstCReqOvrd_C/1 -> switch4/2
  stDstCReqMdl_C/1 -> switch4/1
  switch4/1 -> bus/4  "COM_stDstCReq"
  Sel/4 -> switch4/3  "<MSG06_stDstCReq>"

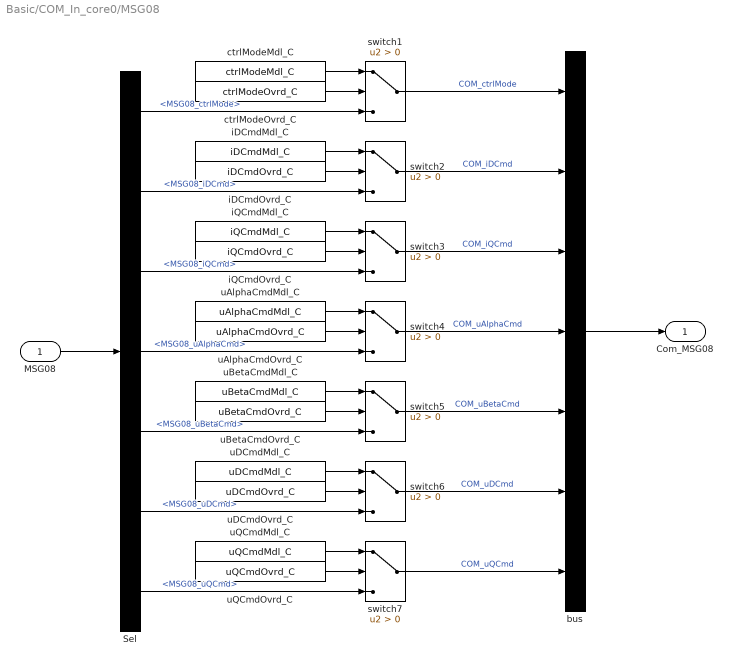
== system Basic/COM_In_core0/MSG08 ==
  MSG08 : Inport
  Sel : BusSelector  OutputSignals=MSG08_ctrlMode,MSG08_iDCmd,MSG08_iQCmd,MSG08_uAlphaCmd,MSG08_uBetaCmd,MSG08_uDCmd,MSG08_uQCmd
  bus : BusCreator  Inputs=7  OutDataTypeStr=Bus: Com_MSG08
  ctrlModeMdl_C : Constant  Value=ctrlModeMdl_C
      mask Display:
      | tmpx = get_param(gcbh,'Value');
      | a= evalin('base',[tmpx,'.Value;']);
      | disp([tmpx,': ',num2str(a)]);
  ctrlModeOvrd_C : Constant  Value=ctrlModeOvrd_C
      mask Display:
      | tmpx = get_param(gcbh,'Value');
      | a= evalin('base',[tmpx,'.Value;']);
      | if a==0
      |     color('blue');
      | else
      |     color('green');
      | end
      | disp([tmpx,': ',num2str(a)]);
  iDCmdMdl_C : Constant  Value=iDCmdMdl_C
      mask Display:
      | tmpx = get_param(gcbh,'Value');
      | a= evalin('base',[tmpx,'.Value;']);
      | disp([tmpx,': ',num2str(a)]);
  iDCmdOvrd_C : Constant  Value=iDCmdOvrd_C
      mask Display:
      | tmpx = get_param(gcbh,'Value');
      | a= evalin('base',[tmpx,'.Value;']);
      | if a==0
      |     color('blue');
      | else
      |     color('green');
      | end
      | disp([tmpx,': ',num2str(a)]);
  iQCmdMdl_C : Constant  Value=iQCmdMdl_C
      mask Display:
      | tmpx = get_param(gcbh,'Value');
      | a= evalin('base',[tmpx,'.Value;']);
      | disp([tmpx,': ',num2str(a)]);
  iQCmdOvrd_C : Constant  Value=iQCmdOvrd_C
      mask Display:
      | tmpx = get_param(gcbh,'Value');
      | a= evalin('base',[tmpx,'.Value;']);
      | if a==0
      |     color('blue');
      | else
      |     color('green');
      | end
      | disp([tmpx,': ',num2str(a)]);
  switch{1..7} (7 alike) : Switch  Criteria=u2 > Threshold  SaturateOnIntegerOverflow=off  InputSameDT=off
  uAlphaCmdMdl_C : Constant  Value=uAlphaCmdMdl_C
      mask Display:
      | tmpx = get_param(gcbh,'Value');
      | a= evalin('base',[tmpx,'.Value;']);
      | disp([tmpx,': ',num2str(a)]);
  uAlphaCmdOvrd_C : Constant  Value=uAlphaCmdOvrd_C
      mask Display:
      | tmpx = get_param(gcbh,'Value');
      | a= evalin('base',[tmpx,'.Value;']);
      | if a==0
      |     color('blue');
      | else
      |     color('green');
      | end
      | disp([tmpx,': ',num2str(a)]);
  uBetaCmdMdl_C : Constant  Value=uBetaCmdMdl_C
      mask Display:
      | tmpx = get_param(gcbh,'Value');
      | a= evalin('base',[tmpx,'.Value;']);
      | disp([tmpx,': ',num2str(a)]);
  uBetaCmdOvrd_C : Constant  Value=uBetaCmdOvrd_C
      mask Display:
      | tmpx = get_param(gcbh,'Value');
      | a= evalin('base',[tmpx,'.Value;']);
      | if a==0
      |     color('blue');
      | else
      |     color('green');
      | end
      | disp([tmpx,': ',num2str(a)]);
  uDCmdMdl_C : Constant  Value=uDCmdMdl_C
      mask Display:
      | tmpx = get_param(gcbh,'Value');
      | a= evalin('base',[tmpx,'.Value;']);
      | disp([tmpx,': ',num2str(a)]);
  uDCmdOvrd_C : Constant  Value=uDCmdOvrd_C
      mask Display:
      | tmpx = get_param(gcbh,'Value');
      | a= evalin('base',[tmpx,'.Value;']);
      | if a==0
      |     color('blue');
      | else
      |     color('green');
      | end
      | disp([tmpx,': ',num2str(a)]);
  uQCmdMdl_C : Constant  Value=uQCmdMdl_C
      mask Display:
      | tmpx = get_param(gcbh,'Value');
      | a= evalin('base',[tmpx,'.Value;']);
      | disp([tmpx,': ',num2str(a)]);
  uQCmdOvrd_C : Constant  Value=uQCmdOvrd_C
      mask Display:
      | tmpx = get_param(gcbh,'Value');
      | a= evalin('base',[tmpx,'.Value;']);
      | if a==0
      |     color('blue');
      | else
      |     color('green');
      | end
      | disp([tmpx,': ',num2str(a)]);
  Com_MSG08 : Outport  VectorParamsAs1DForOutWhenUnconnected=off
  wires:
  MSG08/1 -> Sel/1
  bus/1 -> Com_MSG08/1
  ctrlModeOvrd_C/1 -> switch1/2
  ctrlModeMdl_C/1 -> switch1/1
  switch1/1 -> bus/1  "COM_ctrlMode"
  Sel/1 -> switch1/3  "<MSG08_ctrlMode>"
  iDCmdOvrd_C/1 -> switch2/2
  iDCmdMdl_C/1 -> switch2/1
  switch2/1 -> bus/2  "COM_iDCmd"
  Sel/2 -> switch2/3  "<MSG08_iDCmd>"
  iQCmdOvrd_C/1 -> switch3/2
  iQCmdMdl_C/1 -> switch3/1
  switch3/1 -> bus/3  "COM_iQCmd"
  Sel/3 -> switch3/3  "<MSG08_iQCmd>"
  uAlphaCmdOvrd_C/1 -> switch4/2
  uAlphaCmdMdl_C/1 -> switch4/1
  switch4/1 -> bus/4  "COM_uAlphaCmd"
  Sel/4 -> switch4/3  "<MSG08_uAlphaCmd>"
  uBetaCmdOvrd_C/1 -> switch5/2
  uBetaCmdMdl_C/1 -> switch5/1
  switch5/1 -> bus/5  "COM_uBetaCmd"
  Sel/5 -> switch5/3  "<MSG08_uBetaCmd>"
  uDCmdOvrd_C/1 -> switch6/2
  uDCmdMdl_C/1 -> switch6/1
  switch6/1 -> bus/6  "COM_uDCmd"
  Sel/6 -> switch6/3  "<MSG08_uDCmd>"
  uQCmdOvrd_C/1 -> switch7/2
  uQCmdMdl_C/1 -> switch7/1
  switch7/1 -> bus/7  "COM_uQCmd"
  Sel/7 -> switch7/3  "<MSG08_uQCmd>"

== system Basic/SAQ/cddRt ==
  note: CDDHwMgrST structure is define in structureDefineCdd.m
  CddSt : Inport  OutDataTypeStr=Bus: IO_In_1ms
  buscrt : BusCreator  Inputs=18
  bussel : BusSelector  OutputSignals=flgFO,flgOV,flgSBC,flgUHall,flgVHall,flgWHall,flgUOC,flgVOC,flgWOC,flgHSLV,flgLSLV
  CddSig : Outport  OutDataTypeStr=Bus: Core0_cddRt  VectorParamsAs1DForOutWhenUnconnected=off
  wires:
  buscrt/1 -> CddSig/1
  CddSt/1 -> bussel/1

== system Basic/SAQ/gpiRt ==
  gpiSt : Inport
  busCrt : BusCreator  Inputs=5
  bussel : BusSelector  OutputSignals=KL15,RDYH,RDYL,STL2ASCEN,WAKE
  gpiSig : Outport
  wires:
  gpiSt/1 -> bussel/1
  busCrt/1 -> gpiSig/1

== system Basic/SAQ/vadcRt ==
  vadcSt : Inport
  vadc10ms : Inport  Port=2  OutDataTypeStr=Bus: Core0_ADC_10ms
  Bus Selector : BusSelector  OutputSignals=signal1,signal2
  buscrt : BusCreator  Inputs=22
  bussel : BusSelector  OutputSignals=KL15,RvlRef,KL30
  vadcSig : Outport
  wires:
  vadcSt/1 -> bussel/1
  buscrt/1 -> vadcSig/1
  vadc10ms/1 -> Bus Selector/1
